simulink model "pm4_motor"  (R2017a)
settings: Solver=VariableStepAuto  StartTime=0.0  StopTime=3.0  RelTol=1e-3
libraries: simulink x1
settings Model: Creator=robotica  LastModifiedBy=robotica

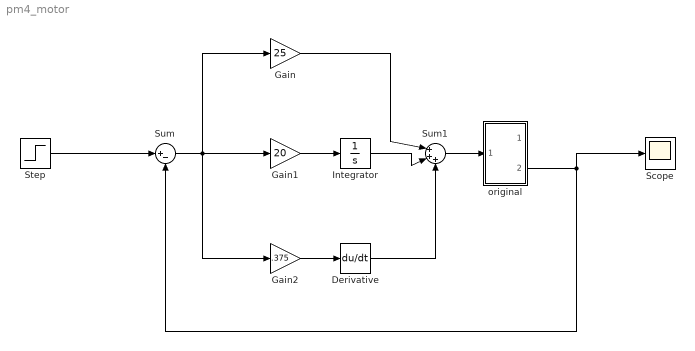
== system pm4_motor ==
  Derivative : Derivative  CoefficientInTFapproximation=0
  Gain : Gain  Gain=25
  Gain1 : Gain  Gain=20
  Gain2 : Gain  Gain=.375
  Integrator : Integrator
  Scope : Scope
  Step : Step  SampleTime=1
  Sum : Sum  Inputs=|+-
  Sum1 : Sum  Inputs=|+++
  original : Subsystem
  wires:
  Step/1 -> Sum/1
  original/2(clean) -> Sum/2, Scope/1
  Gain/1 -> Sum1/1
  Sum/1 -> Gain2/1, Gain/1, Gain1/1
  Gain2/1 -> Derivative/1
  Gain1/1 -> Integrator/1
  Sum1/1 -> original/1(signal)
  Integrator/1 -> Sum1/2
  Derivative/1 -> Sum1/3

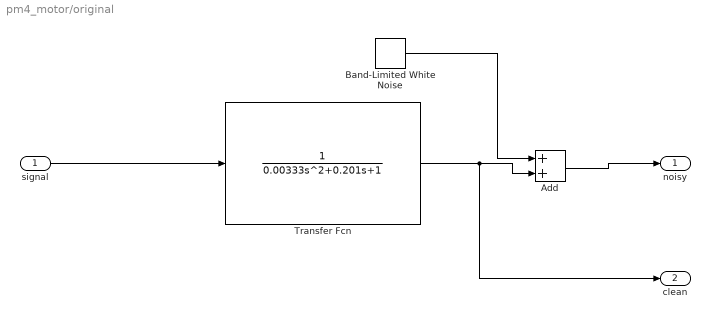
== system pm4_motor/original ==
  signal : Inport
  Add : Sum
  Band-Limited White Noise : simulink/Sources/Band-Limited White Noise  Cov=[0.0000001]  Ts=0.001  seed=[23341]
  Transfer Fcn : TransferFcn  Denominator=[0.00333 0.201 1]
  noisy : Outport
  clean : Outport  Port=2
  wires:
  Transfer Fcn/1 -> clean/1, Add/2
  Band-Limited White Noise/1 -> Add/1
  Add/1 -> noisy/1
  signal/1 -> Transfer Fcn/1
